simulink model "rlKinovaBallBalance_lags"  (R2024a)
settings: Solver=ode15s  StartTime=0.0  StopTime=inf  MaxStep=0.005  RelTol=1e-4  AbsTol=1e-4
values from neighbouring files (symbols this model uses):
  abs_max_torque_U = [6, 0.70, 2.12, 0.505]    [kinova_params.m]
  g = 3.71    [kinova_params.m]
  max_angular_vel = 2.0    (= 2)    [kinova_params.m]
  max_linear_vel = 0.6    [kinova_params.m]
  max_torque = [1.6; 0.6; 0.9; 0.5]    [kinova_params.m]
  max_torque_PD = [2.5; 0.6; 0.6; 0.3]    [kinova_params.m]
  R1_q0 = 0    [kinova_params.m]
  R2_q0 = deg2rad(20)    [kinova_params.m]
  R3_q0 = 0    [kinova_params.m]
  R4_q0 = deg2rad(135)    [kinova_params.m]
  R5_q0 = 0    [kinova_params.m]
  R6_q0 = deg2rad(-65)    [kinova_params.m]
  R7_q0 = deg2rad(-90)    [kinova_params.m]
  rlEpisodeFinalTime = 21    [kinova_params.m]
  rlStartTime = 0    [kinova_params.m]
  rlTimeStep = 0.01    [kinova_params.m]
  U0 = [-5.75, 0.10, -1.3, 0.0]    [kinova_params.m]
undefined symbols (not defined in the file or in its folder): Control, fluent0, L1, L2, L3, LS1, LS3, plate, R1, R2, R3, Rover, rover_path, RS1, RS3, Ts, vessel, X, Y, Z
libraries: sm_lib x251, nesl_utility x110, fl_lib x85, nesl_utility_internal x34, sdl_lib x20, simulink x16, ee_lib x10, mars_rover_lib x6, slpidlib x2, batteryecm_lib x2, robotalgslib x1, rllib x1
(part 13 of 13)

== matlab function rlKinovaBallBalance_lags/Kinova Ball Balance/Control/Chassis Control/Chassis Velocity To Wheel Speed ==
  data: vTarget input; steer_ang input; A3_ROC input; L3_ROC input; R3_ROC input; wL1 output; wheel_r input; wL2 output; wL3 output; L input; wR1 output; wR2 output; wR3 output
function [wL1,wL2,wL3, wR1,wR2,wR3] = ...
    fcn(vTarget,steer_ang,A3_ROC,L3_ROC,R3_ROC,wheel_r,L)
% Function to compute wheel speed from a desired linear velocity and
% desired path.

if any(abs(steer_ang) > 0)

    wL1 = (vTarget/wheel_r)*sqrt(L3_ROC^2 + L^2)/A3_ROC;
    wL2 = vTarget * L3_ROC/(A3_ROC*wheel_r);
    wL3 = (vTarget/wheel_r)*sqrt(L3_ROC^2 + L^2)/A3_ROC;
    wR1 = (vTarget/wheel_r)*sqrt(R3_ROC^2 + L^2)/A3_ROC;
    wR2 = vTarget * R3_ROC/(A3_ROC*wheel_r);
    wR3 = (vTarget/wheel_r)*sqrt(R3_ROC^2 + L^2)/A3_ROC;

else
    wL1 = vTarget / wheel_r;
    wL2 = vTarget / wheel_r;
    wL3 = vTarget / wheel_r;
    wR1 = vTarget / wheel_r;
    wR2 = vTarget / wheel_r;
    wR3 = vTarget / wheel_r;
end

end

== matlab function rlKinovaBallBalance_lags/Kinova Ball Balance/Control/Chassis Control/Target Dir To Bicycle Steer Angle/Rad2Deg ==
  data: u input; y output
function y = fcn(u)
y = rad2deg(u);

== matlab function rlKinovaBallBalance_lags/Kinova Ball Balance/Control/Chassis Control/Target Direction and Speed/Trapezoidal Vel Profile ==
  data: t input; startTime input; accel input; deaccelStartTime input; linVel input; lin_Vel_out output
function lin_Vel_out = fcn(t,startTime,accel,deaccelStartTime,linVel)
% Function to create a trapezoidal profile for rover's desired linear
% velocity

t2 = linVel/accel + startTime;
t3 = deaccelStartTime + 0.2;
tf = linVel/accel + t3;

if t>=startTime && t<t2 
    lin_Vel_out = accel*(t-startTime);

elseif t>=t2 && t < t3 
    lin_Vel_out = linVel;

elseif t>= t3 && t < tf 
    lin_Vel_out = linVel-accel*(t-t3);

else
    lin_Vel_out = 0;    
end


end
